simulink library "Nacelle_Lib"  (Simulink 7.9)
settings: Solver=ode45  StartTime=0.0  StopTime=10.0  RelTol=1e-3
undefined symbols (not defined in the file): WT_Params
libraries: mblibv1 x2, Geartrain_Lib x1, Generator_Lib x1, Hub_Axis_Lib x1, Pitch_System_Lib x1, Yaw_System_Lib x1
Description:
  | Copyright 2011 MathWorks, Inc.
settings Model: Creator=smiller  LastModifiedBy=smiller

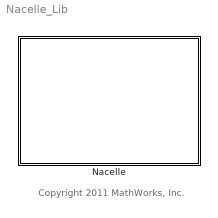
== system Nacelle_Lib ==
  note: Copyright 2011 MathWorks, Inc.
  Nacelle : Subsystem  RequirementInfo={'other' 'Wind_Turbine_Requirements.doc' '@Simulink_requirement_item_2' 'true' 'Yaw Actuation Requirements' '' } %GIDa_4b2bb41f_4c80_4421_bc27_2f83bb871036
      mask Display:
      | image(imread('Nacelle_IMAGE.jpg'));
      | port_label('RConn',1,'YC');
      | port_label('RConn',2,'Br');
      | port_label('RConn',3,'G');
      | port_label('RConn',4,'T');
      | port_label('RConn',5,'GrVa');
      | port_label('RConn',6,'GrVb');
      | port_label('RConn',7,'GrVc');
      | port_label('LConn',1,'PC');
      | port_label('LConn',2,'B1');
      | port_label('LConn',3,'BPA1');
      | port_label('LConn',4,'B2');
      | port_label('LConn',5,'BPA2');
      | port_label('LConn',6,'B3');
      | port_label('LConn',7,'BPA3');

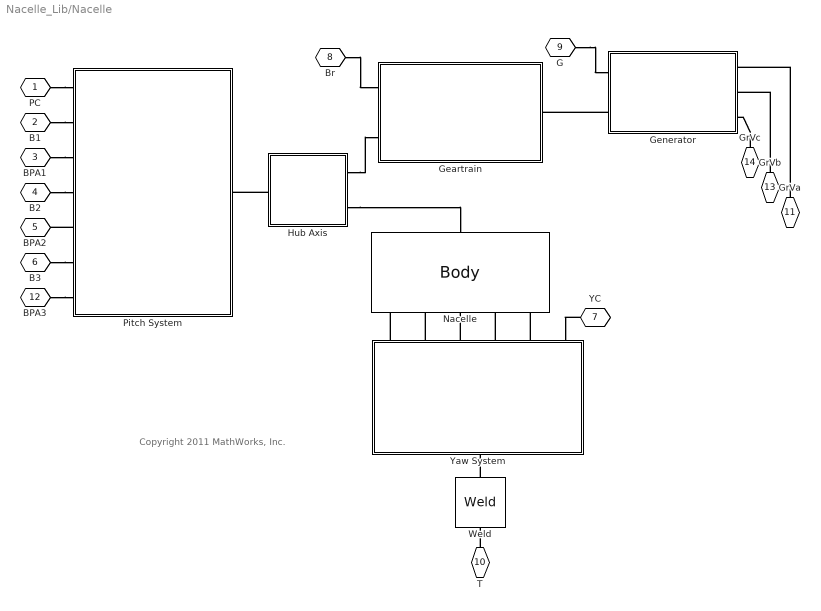
== system Nacelle_Lib/Nacelle ==
  note: Copyright 2011 MathWorks, Inc.
  Geartrain : Subsystem  BlockChoice=Ideal
      settings: AttributesFormatString=%<BlockChoice>  TemplateBlock=Geartrain_Lib/Geartrain  MemberBlocks=Empty,Ideal
  Generator : Subsystem  BlockChoice=Simple
      settings: AttributesFormatString=%<BlockChoice>  TemplateBlock=Generator_Lib/Generator  MemberBlocks=Full,Simple
  Hub Axis : Subsystem  BlockChoice=Rotate
      settings: AttributesFormatString=%<BlockChoice>  TemplateBlock=Hub_Axis_Lib/Hub Axis  MemberBlocks=Locked,Rotate
  Nacelle : mblibv1/Bodies/Body  PhysicalDomain=mechanical  SubClassName=Unknown  LeftPortType=workingframe  RightPortType=workingframe  LConnTagsString=CS2  RConnTagsString=CS5|CS7|CS3|CS9|CS11  UpdateFromCAD=off  DialogClass=MechanicalBodyBlock  Mass=WT_Params.Nacelle.mass  MassUnits=kg  InertiaUnits=kg*m^2  Inertia=WT_Params.Nacelle.inertia  Shape=Cylinder  ShapeDims=[1 1]  ShapeUnits=m  ShapeUse=false  Density=1  DensityUnits=kg/m^3  DensityUse=false  GraphicsMode=MACHINE_DEFAULT  BodyColorSelMode=COLORPALETTE  BodyColor=[1 1 1]  AttachedToCS=CG  CG=Left$CG$[-WT_Params.Nacelle.CG_Offset.x WT_Params.Nacelle.CG_Offset.y 0]$CS1$CS1$m$[0 0 0]$Euler X-Y-Z$deg$CS3$false$none  WorkingFrames=Left$CS1$[WT_Params.Nacelle.Yaw_Ctr_Offset.x WT_Params.Nacelle.Yaw_Ctr_Offset.y 0]$CS3$CS3$m$[0 0 0]$Euler X-Y-Z$deg$CS3$false$none#Left$CS2$[-WT_Params.Nacelle.length 0 0]$CS1$CS1$m$[0 0 0]$Euler X-Y-Z$deg$CS3$true$none#Left$CS4$[0 0 0]$CS3$CS3$m$[0 45 0]$Euler X-Y-Z$deg$CS1$false$none#Right$CS5$[WT_Params.Yaw_Actuator.yaw_ring_diameter/2+WT_Params.Yaw_Actuator.yaw_gear_diameter/2 0 0]$CS4$CS4$m$[0 0 0]$Euler X-Y-Z$deg$CS1$true$none#Left$CS6$[0 0 0]$CS3$CS3$m$[0 135 0]$Euler X-Y-Z$deg$CS1$false$none#Right$CS7$[WT_Params.Yaw_Actuator.yaw_ring_diameter/2+WT_Params.Yaw_Actuator.yaw_gear_diameter/2 0 0]$CS6$CS6$m$[0 0 0]$Euler X-Y-Z$deg$CS1$true$none#Right$CS3$[0 0 0]$Adjoining$Adjoining$m$[0 0 0]$Euler X-Y-Z$deg$Adjoining$true$none#Left$CS8$[0 0 0]$CS3$CS3$m$[0 225 0]$Euler X-Y-Z$deg$CS1$false$none#Right$CS9$[WT_Params.Yaw_Actuator.yaw_ring_diameter/2+WT_Params.Yaw_Actuator.yaw_gear_diameter/2 0 0]$CS8$CS8$m$[0 0 0]$Euler X-Y-Z$deg$CS1$true$none#Left$CS10$[0 0 0]$CS3$CS3$m$[0 315 0]$Euler X-Y-Z$deg$CS1$false$none#Right$CS11$[WT_Params.Yaw_Actuator.yaw_ring_diameter/2+WT_Params.Yaw_Actuator.yaw_gear_diameter/2 0 0]$CS10$CS10$m$[0 0 0]$Euler X-Y-Z$deg$CS1$true$none  CGPos=[-WT_Params.Nacelle.CG_Offset.x WT_Params.Nacelle.CG_Offset.y 0]  CGRot=[0 0 0]  CS0Pos=[]  CS0Rot=[]  CS1Pos=[WT_Params.Nacelle.Yaw_Ctr_Offset.x WT_Params.Nacelle.Yaw_Ctr_Offset.y 0]  CS1Rot=[0 0 0]  CS2Pos=[-WT_Params.Nacelle.length 0 0]  CS2Rot=[0 0 0]  CS3Pos=[0 0 0]  CS3Rot=[0 0 0]  CS4Pos=[0 0 0]  CS4Rot=[0 45 0]  CS5Pos=[WT_Params.Yaw_Actuator.yaw_ring_diameter/2+WT_Params.Yaw_Actuator.yaw_gear_diameter/2 0 0]  CS5Rot=[0 0 0]  CS6Pos=[0 0 0]  CS6Rot=[0 135 0]  CS7Pos=[WT_Params.Yaw_Actuator.yaw_ring_diameter/2+WT_Params.Yaw_Actuator.yaw_gear_diameter/2 0 0]  CS7Rot=[0 0 0]  CS8Pos=[0 0 0]  CS8Rot=[0 225 0]  CS9Pos=[WT_Params.Yaw_Actuator.yaw_ring_diameter/2+WT_Params.Yaw_Actuator.yaw_gear_diameter/2 0 0]  CS9Rot=[0 0 0]  CS10Pos=[0 0 0]  CS10Rot=[0 315 0]  CS11Pos=[WT_Params.Yaw_Actuator.yaw_ring_diameter/2+WT_Params.Yaw_Actuator.yaw_gear_diameter/2 0 0]  CS11Rot=[0 0 0]  CS12Pos=[]  CS12Rot=[]  CS13Pos=[]  CS13Rot=[]  CS14Pos=[]  CS14Rot=[]  CS15Pos=[]  CS15Rot=[]  CS16Pos=[]  CS16Rot=[]  CS17Pos=[]  CS17Rot=[]  CS18Pos=[]  CS18Rot=[]  CS19Pos=[]  CS19Rot=[]  CS20Pos=[]  CS20Rot=[]
  Pitch System : Subsystem  BlockChoice=Ideal
      settings: AttributesFormatString=%<BlockChoice>  TemplateBlock=Pitch_System_Lib/Pitch System  MemberBlocks=Hydraulic,Ideal,Locked
  Weld : mblibv1/Joints/Weld  LConnTagsString=__newl0  RConnTagsString=__newr0  UpdateFromCAD=off  NumSAPorts=0  CutJoint=off  MarkAsCut=off  Primitives=weld  PrimitiveProps=W$WORLD$[0 0 0]$weld  DialogClass=JointBlock  WAxis=[0 0 0]
  Yaw System : Subsystem  BlockChoice=Ideal Actuator
      settings: AttributesFormatString=%<BlockChoice>  TemplateBlock=Yaw_System_Lib/Yaw System  MemberBlocks=Ideal Actuator,Ideal Motor,Locked,Servomotor
  PC : PMIOPort  Tag=PMCPort  Port=1  Side=Left
  B1 : PMIOPort  Tag=PMCPort  Port=2  Side=Left
  BPA1 : PMIOPort  Tag=PMCPort  Port=3  Side=Left
  B2 : PMIOPort  Tag=PMCPort  Port=4  Side=Left
  BPA2 : PMIOPort  Tag=PMCPort  Port=5  Side=Left
  B3 : PMIOPort  Tag=PMCPort  Port=6  Side=Left
  YC : PMIOPort  Tag=PMCPort  Port=7  Side=Right
  Br : PMIOPort  Tag=PMCPort  Port=8  Side=Right
  G : PMIOPort  Tag=PMCPort  Port=9  Side=Right
  T : PMIOPort  Tag=PMCPort  Port=10  Side=Right
  GrVa : PMIOPort  Tag=PMCPort  Port=11  Side=Right
  BPA3 : PMIOPort  Tag=PMCPort  Port=12  Side=Left
  GrVb : PMIOPort  Tag=PMCPort  Port=13  Side=Right
  GrVc : PMIOPort  Tag=PMCPort  Port=14  Side=Right
  connections:
  Hub Axis/RConn1 -- Geartrain/LConn2
  YC/RConn1 -- Yaw System/RConn6
  Weld/RConn1 -- Yaw System/LConn1
  Yaw System/RConn5 -- Nacelle/RConn5
  Yaw System/RConn4 -- Nacelle/RConn4
  Yaw System/RConn2 -- Nacelle/RConn2
  Yaw System/RConn1 -- Nacelle/RConn1
  Yaw System/RConn3 -- Nacelle/RConn3
  Hub Axis/RConn2 -- Nacelle/LConn1
  T/RConn1 -- Weld/LConn1
  B1/RConn1 -- Pitch System/LConn2
  B2/RConn1 -- Pitch System/LConn4
  PC/RConn1 -- Pitch System/LConn1
  GrVa/RConn1 -- Generator/RConn1
  G/RConn1 -- Generator/LConn1
  Generator/LConn2 -- Geartrain/RConn1
  Hub Axis/LConn1 -- Pitch System/RConn1
  B3/RConn1 -- Pitch System/LConn6
  BPA1/RConn1 -- Pitch System/LConn3
  Pitch System/LConn5 -- BPA2/RConn1
  BPA3/RConn1 -- Pitch System/LConn7
  Br/RConn1 -- Geartrain/LConn1
  GrVb/RConn1 -- Generator/RConn2
  GrVc/RConn1 -- Generator/RConn3

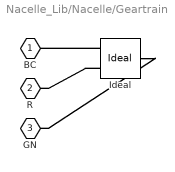
== system Nacelle_Lib/Nacelle/Geartrain ==
  Ideal : Geartrain_Lib/Ideal  SystemSampleTime=-1
  BC : PMIOPort  Port=1  Side=Left
  R : PMIOPort  Port=2  Side=Left
  GN : PMIOPort  Port=3  Side=Right
  connections:
  Ideal/LConn1 -- BC/RConn1
  Ideal/LConn2 -- R/RConn1
  Ideal/RConn1 -- GN/RConn1

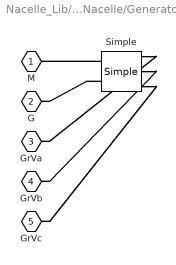
== system Nacelle_Lib/Nacelle/Generator ==
  Simple : Generator_Lib/Simple  SystemSampleTime=-1
  M : PMIOPort  Port=1  Side=Left
  G : PMIOPort  Port=2  Side=Left
  GrVa : PMIOPort  Port=3  Side=Right
  GrVb : PMIOPort  Port=4  Side=Right
  GrVc : PMIOPort  Port=5  Side=Right
  connections:
  Simple/LConn1 -- M/RConn1
  Simple/LConn2 -- G/RConn1
  Simple/RConn1 -- GrVa/RConn1
  Simple/RConn2 -- GrVb/RConn1
  Simple/RConn3 -- GrVc/RConn1

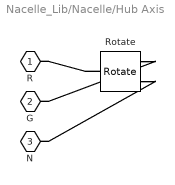
== system Nacelle_Lib/Nacelle/Hub Axis ==
  Rotate : Hub_Axis_Lib/Rotate  SystemSampleTime=-1
  R : PMIOPort  Port=1  Side=Left
  G : PMIOPort  Port=2  Side=Right
  N : PMIOPort  Port=3  Side=Right
  connections:
  Rotate/LConn1 -- R/RConn1
  Rotate/RConn1 -- G/RConn1
  Rotate/RConn2 -- N/RConn1

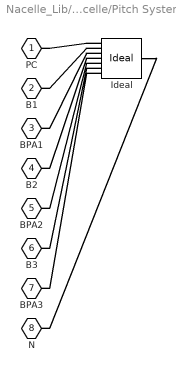
== system Nacelle_Lib/Nacelle/Pitch System ==
  Ideal : Pitch_System_Lib/Ideal  SystemSampleTime=-1
  PC : PMIOPort  Port=1  Side=Left
  B1 : PMIOPort  Port=2  Side=Left
  BPA1 : PMIOPort  Port=3  Side=Left
  B2 : PMIOPort  Port=4  Side=Left
  BPA2 : PMIOPort  Port=5  Side=Left
  B3 : PMIOPort  Port=6  Side=Left
  BPA3 : PMIOPort  Port=7  Side=Left
  N : PMIOPort  Port=8  Side=Right
  connections:
  Ideal/LConn1 -- PC/RConn1
  Ideal/LConn2 -- B1/RConn1
  Ideal/LConn3 -- BPA1/RConn1
  Ideal/LConn4 -- B2/RConn1
  Ideal/LConn5 -- BPA2/RConn1
  Ideal/LConn6 -- B3/RConn1
  Ideal/LConn7 -- BPA3/RConn1
  Ideal/RConn1 -- N/RConn1

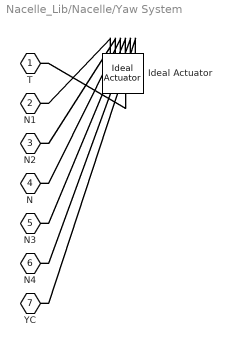
== system Nacelle_Lib/Nacelle/Yaw System ==
  Ideal Actuator : Yaw_System_Lib/Ideal Actuator  SystemSampleTime=-1
  T : PMIOPort  Port=1  Side=Left
  N1 : PMIOPort  Port=2  Side=Right
  N2 : PMIOPort  Port=3  Side=Right
  N : PMIOPort  Port=4  Side=Right
  N3 : PMIOPort  Port=5  Side=Right
  N4 : PMIOPort  Port=6  Side=Right
  YC : PMIOPort  Port=7  Side=Right
  connections:
  Ideal Actuator/LConn1 -- T/RConn1
  Ideal Actuator/RConn1 -- N1/RConn1
  Ideal Actuator/RConn2 -- N2/RConn1
  Ideal Actuator/RConn3 -- N/RConn1
  Ideal Actuator/RConn4 -- N3/RConn1
  Ideal Actuator/RConn5 -- N4/RConn1
  Ideal Actuator/RConn6 -- YC/RConn1
